simulink model "Autopilot_pwa_mdl"  (R2018b)
settings: Solver=VariableStepAuto  StartTime=0.0  StopTime=3  MaxStep=0.01  RelTol=1e-3
values from neighbouring files (symbols this model uses):
  ns = order(pdG)    [lpvctrl.m]    (also in lpvctrl_2.m = size(akh,1); pcss_Sfunction.m = order(sys))
  nu = length(pdG.InputGroup.ctrl)    [lpvctrl.m]    (also in lpvctrl_2.m; test_lpvanalysis.m = 0:10)
  ny = 0    [lft_pass.m]    (also in lft_pgss.m; lft_ppss.m; lpvctrl.m = length(pdG.OutputGroup.meas); lpvctrl_2.m = length(pdG.OutputGroup.meas))
  pdK = ppss(pdk,pdG.parset,                         'OutputName',pdG.OutputName(pdG.OutputGroup.meas),                         'InputName',pdG.InputName(pdG.InputGroup.ctrl))    [lpvctrl.m]    (also in lpvctrl_2.m)
libraries: cstblocks x4, simulink x1
settings Model: Creator=ferna  LastModifiedBy=ferna

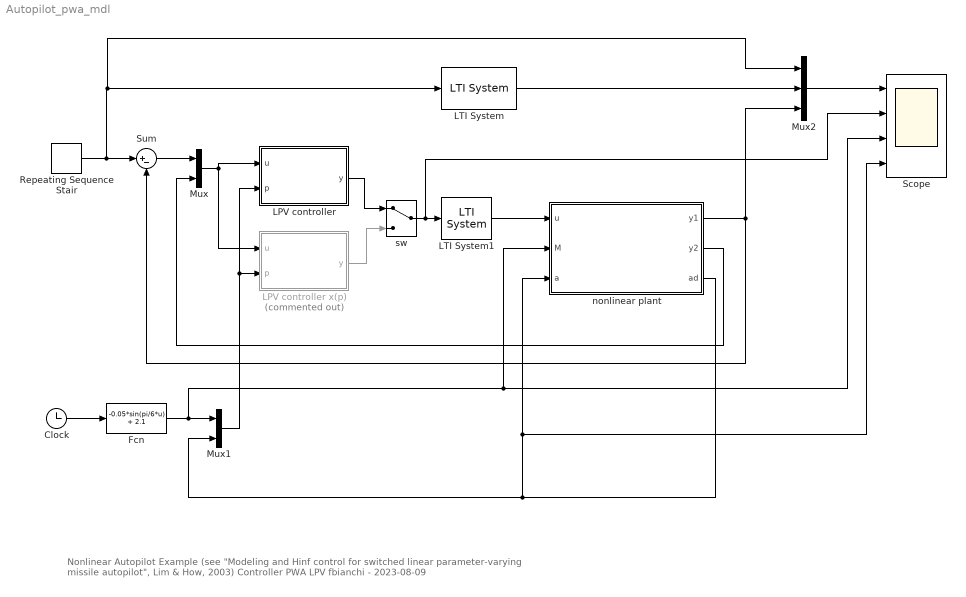
== system Autopilot_pwa_mdl ==
  note: Nonlinear Autopilot Example (see "Modeling and Hinf control for switched linear parameter-varying missile autopilot", Lim & How, 2003)
      | Controller PWA LPV
      | fbianchi - 2023-08-09
  Clock : Clock
  Fcn : Fcn  Expr=-0.05*sin(pi/6*u) + 2.1
  LPV controller : Subsystem  mask{pdG=pdK, x0=0}
      mask prompts: pdG "LPV Model (pass, ppss, pgss)"; x0 "Initial conditions"
      mask init:
      | % model dimensions
      | [ny,nu,ns,np,nv] = size(pdG);
      | 
      | % interpolation 
      | type = class(pdG);
      | switch type
      |     case 'pass'
      |         fcn = [];
      |         
      |     case 'pgss'
      |         fcn = pdg.parfcn;
      |         
      |     case 'ppss'
      |         fcn = pdG.parset;
      | end
      | 
      | % model matrices
      | M = [pdG.A pdG.B;
      |      pdG.C pdG.D];
      | Mdata = reshape(M,(ns+ny)*(ns+nu),nv,1);
      mask Display:
      | disp('LPV model')
      | port_label('input', 1, 'u')
      | port_label('input', 2, 'p')
      | port_label('output', 1, 'y')
  LPV controller x(p) : Subsystem  Commented=on  mask{pdK=pdK, x0=0}
      mask prompts: pdK "Controller (pcss)"; x0 "Initial conditions"
      mask init:
      | % model dimensions
      | [ny,nu,ns,np,nv] = size(pdK.ctrller);
      | 
      | % controller data
      | % interpolation 
      | type = class(pdK.ctrller);
      | switch type
      |     case 'pass'
      |         fcn = [];
      |         
      |     case 'pgss'
      |         fcn = pdK.ctrller.parfcn;
      |         
      |     case 'ppss'
      |         fcn = pdK.ctrller.parset;
      | end
      | 
      | % controller variables at p
      | K = [pdK.ctrller.A pdK.ctrller.B;
      |      pdK.ctrller.C pdK.ctrller.D];
      | Kdata = reshape(K,(ns+ny)*(ns+nu),nv,1);
      | 
      | % Lyapunov function at par
      | flagX = isnumeric(pdK.xFcn);
      | flagY = isnumeric(pdK.yFcn);
      | if (flagX == 0) && (flagY == 0)
      |     Ydata = reshape(pdK.yFcn.D,ns*ns,nv,1);
      |     Xdata = reshape(pdK.xFcn.D,ns*ns,nv,1);
      |     
      | elseif (flagX == 1) && (flagY == 0)
      |     Xdata = pdK.xFcn;
      |     Ydata = reshape(pdK.yFcn.D,ns*ns,nv,1);
      |     
      | elseif (flagX == 0) && (flagY == 1)
      |     Xdata = reshape(pdK.xFcn.D,ns*ns,nv,1);
      |     Ydata = pdK.yFcn;
      |     
      | end
      |                
      | % augmented plant matrices
      | Adata  = reshape(pdK.plant.A,ns*ns,nv,1);
      | b2 = pdK.plant.B(:,:,1);
      | c2 = pdK.plant.C(:,:,1);
      mask Display:
      | disp('pcss ctrller')
      | port_label('input', 1, 'u')
      | port_label('input', 2, 'p')
      | port_label('output', 1, 'y')
  LTI System : cstblocks/LTI System  sys=Wref  IC=[]
  LTI System1 : cstblocks/LTI System  sys=Act  IC=[]
  Mux : Mux  Inputs=2
  Mux1 : Mux  Inputs=2
  Mux2 : Mux  Inputs=3
  Repeating Sequence Stair : simulink/Sources/Repeating Sequence Stair  OutValues=[10 -15 0 0].'  tsamp=1  OutMin=[]  OutMax=[]  OutDataTypeStr=double  OutputDataTypeScalingMode=double  OutDataType=fixdt(0,8)  ConRadixGroup=Best Precision: Vector-wise  OutScaling=2^-12
  Scope : Scope  NumInputPorts=4
  Sum : Sum  Inputs=|+-
  nonlinear plant : Subsystem
  sw : ManualSwitch
  wires:
  LTI System1/1 -> nonlinear plant/1(u)
  Mux/1 -> LPV controller/1("u "), LPV controller x(p)/1("u ")
  Sum/1 -> Mux/1
  nonlinear plant/2(y2) -> Mux/2
  nonlinear plant/1(y1) -> Mux2/3, Sum/2
  Clock/1 -> Fcn/1
  Fcn/1 -> nonlinear plant/2(M), Scope/3, Mux1/1
  Mux1/1 -> LPV controller/2(p), LPV controller x(p)/2(p)
  Repeating Sequence Stair/1 -> LTI System/1, Mux2/1, Sum/1
  Mux2/1 -> Scope/1
  LTI System/1 -> Mux2/2
  nonlinear plant/3(ad) -> Mux1/2, nonlinear plant/3(a), Scope/4
  LPV controller/1(y) -> sw/1
  sw/1 -> Scope/2, LTI System1/1
  LPV controller x(p)/1(y) -> sw/2

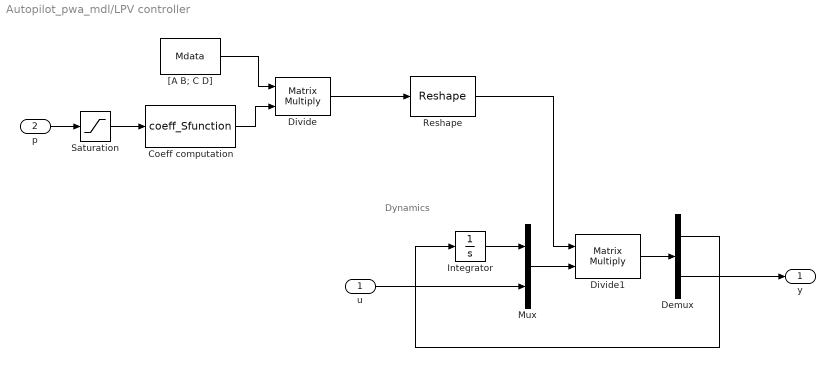
== system Autopilot_pwa_mdl/LPV controller ==
  note: Dynamics
  "u " : Inport
  p : Inport  Port=2
  Coeff computation : M-S-Function  FunctionName=coeff_Sfunction  Parameters=np, nv, fcn, type
  Demux : Demux  Outputs=[ns, ny]
  Divide : Product  Inputs=**  Multiplication=Matrix(*)
  Divide1 : Product  Inputs=**  Multiplication=Matrix(*)
  Integrator : Integrator
  Mux : Mux  Inputs=[ns, nu]
  Reshape : Reshape  OutputDimensionality=Customize  OutputDimensions=[ns+ny, ns+nu, 1]
  Saturation : Saturate  UpperLimit=pdK.parset.range(:,2)  LowerLimit=pdK.parset.range(:,1)
  "[A B; C D]" : Constant  Value=Mdata  VectorParams1D=off
  y : Outport
  wires:
  Divide/1 -> Reshape/1
  p/1 -> Saturation/1
  Saturation/1 -> Coeff computation/1
  Reshape/1 -> Divide1/1
  Mux/1 -> Divide1/2
  Divide1/1 -> Demux/1
  Demux/2 -> y/1
  Demux/1 -> Integrator/1
  Integrator/1 -> Mux/1
  "u "/1 -> Mux/2
  Coeff computation/1 -> Divide/2
  "[A B; C D]"/1 -> Divide/1

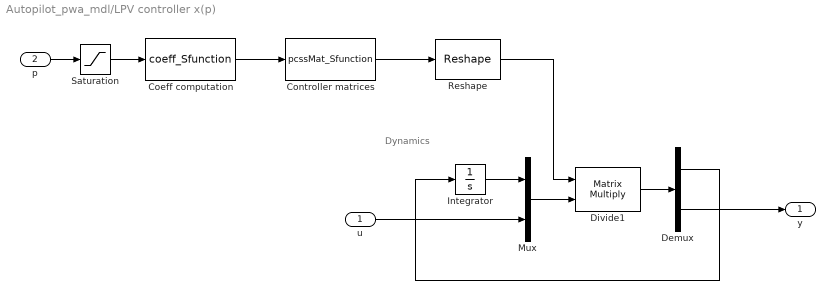
== system Autopilot_pwa_mdl/LPV controller x(p) ==
  note: Dynamics
  "u " : Inport
  p : Inport  Port=2
  Coeff computation : M-S-Function  FunctionName=coeff_Sfunction  Parameters=np, nv, fcn, type
  Controller matrices : M-S-Function  FunctionName=pcssMat_Sfunction  Parameters=Kdata, Xdata, Ydata, Adata, b2, c2, ns, ny, nu, nv, flagX, flagY
  Demux : Demux  Outputs=[ns, ny]
  Divide1 : Product  Inputs=**  Multiplication=Matrix(*)
  Integrator : Integrator
  Mux : Mux  Inputs=[ns, nu]
  Reshape : Reshape  OutputDimensionality=Customize  OutputDimensions=[ns+ny, ns+nu, 1]
  Saturation : Saturate  UpperLimit=pdK.parset.range(:,2)  LowerLimit=pdK.parset.range(:,1)
  y : Outport
  wires:
  "u "/1 -> Mux/2
  Integrator/1 -> Mux/1
  Demux/1 -> Integrator/1
  Demux/2 -> y/1
  Divide1/1 -> Demux/1
  Mux/1 -> Divide1/2
  Reshape/1 -> Divide1/1
  Saturation/1 -> Coeff computation/1
  p/1 -> Saturation/1
  Coeff computation/1 -> Controller matrices/1
  Controller matrices/1 -> Reshape/1

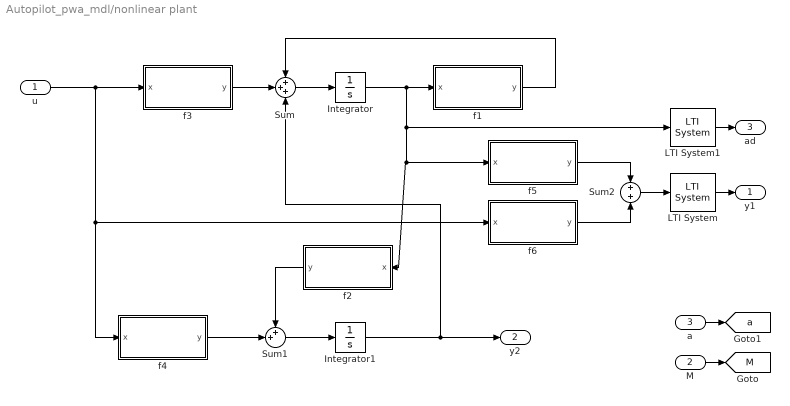
== system Autopilot_pwa_mdl/nonlinear plant ==
  u : Inport
  M : Inport  Port=2
  a : Inport  Port=3
  Integrator : Integrator
  Integrator1 : Integrator
  LTI System : cstblocks/LTI System  sys=F  IC=[]
  LTI System1 : cstblocks/LTI System  sys=F  IC=[]
  Sum : Sum  Inputs=+++
  Sum1 : Sum  Inputs=++|
  Sum2 : Sum
  f1 : Subsystem
  f2 : Subsystem
  f3 : Subsystem
  f4 : Subsystem
  f5 : Subsystem
  f6 : Subsystem
  y1 : Outport
  y2 : Outport  Port=2
  ad : Outport  Port=3
  tag scope: M=global, a=global
  wires:
  a/1 -> [a]
  f6/1(y) -> Sum2/2
  M/1 -> [M]
  f1/1(y) -> Sum/1
  f3/1(y) -> Sum/2
  Integrator/1 -> f2/1(x), f5/1(x), LTI System1/1, f1/1(x)
  Integrator1/1 -> Sum/3, y2/1
  f5/1(y) -> Sum2/1
  Sum/1 -> Integrator/1
  Sum2/1 -> LTI System/1
  u/1 -> f6/1(x), f4/1(x), f3/1(x)
  LTI System/1 -> y1/1
  LTI System1/1 -> ad/1
  Sum1/1 -> Integrator1/1
  f4/1(y) -> Sum1/2
  f2/1(y) -> Sum1/1

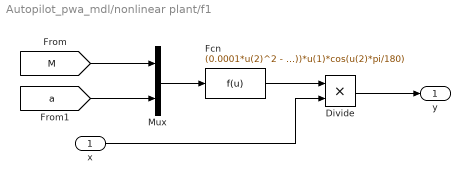
== system Autopilot_pwa_mdl/nonlinear plant/f1 ==
  x : Inport
  Divide : Product  Inputs=**
  Fcn : Fcn  Expr=(0.0001*u(2)^2 - 0.0112*abs(u(2)) - 0.2010*(2 - u(1)/3))*u(1)*cos(u(2)*pi/180)
  Mux : Mux  Inputs=2
  y : Outport
  wires:
  [a] -> Mux/2
  Mux/1 -> Fcn/1
  [M] -> Mux/1
  Fcn/1 -> Divide/1
  Divide/1 -> y/1
  x/1 -> Divide/2

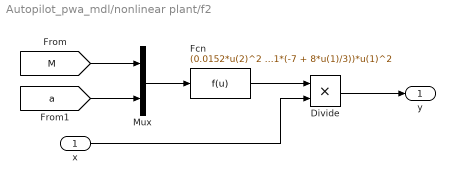
== system Autopilot_pwa_mdl/nonlinear plant/f2 ==
  x : Inport
  Divide : Product  Inputs=**
  Fcn : Fcn  Expr=(0.0152*u(2)^2 - 1.3765*abs(u(2)) + 3.6001*(-7 + 8*u(1)/3))*u(1)^2
  Mux : Mux  Inputs=2
  y : Outport
  wires:
  x/1 -> Divide/2
  Divide/1 -> y/1
  Fcn/1 -> Divide/1
  [M] -> Mux/1
  Mux/1 -> Fcn/1
  [a] -> Mux/2

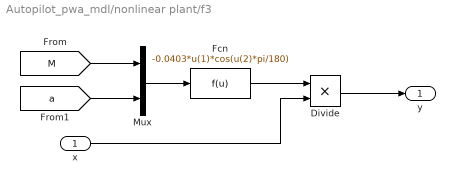
== system Autopilot_pwa_mdl/nonlinear plant/f3 ==
  x : Inport
  Divide : Product  Inputs=**
  Fcn : Fcn  Expr=-0.0403*u(1)*cos(u(2)*pi/180)
  Mux : Mux  Inputs=2
  y : Outport
  wires:
  Mux/1 -> Fcn/1
  Fcn/1 -> Divide/1
  Divide/1 -> y/1
  x/1 -> Divide/2
  [a] -> Mux/2
  [M] -> Mux/1

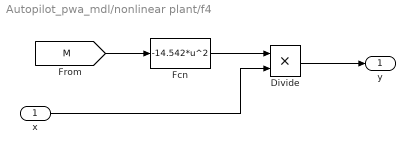
== system Autopilot_pwa_mdl/nonlinear plant/f4 ==
  x : Inport
  Divide : Product  Inputs=**
  Fcn : Fcn  Expr=-14.542*u^2
  y : Outport
  wires:
  x/1 -> Divide/2
  Divide/1 -> y/1
  Fcn/1 -> Divide/1
  [M] -> Fcn/1

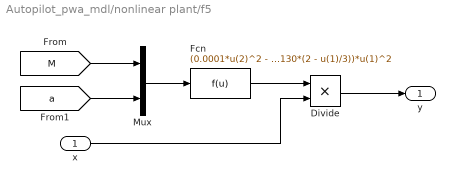
== system Autopilot_pwa_mdl/nonlinear plant/f5 ==
  x : Inport
  Divide : Product  Inputs=**
  Fcn : Fcn  Expr=(0.0001*u(2)^2 - 0.0063*abs(u(2)) - 0.1130*(2 - u(1)/3))*u(1)^2
  Mux : Mux  Inputs=2
  y : Outport
  wires:
  Mux/1 -> Fcn/1
  Fcn/1 -> Divide/1
  Divide/1 -> y/1
  x/1 -> Divide/2
  [a] -> Mux/2
  [M] -> Mux/1

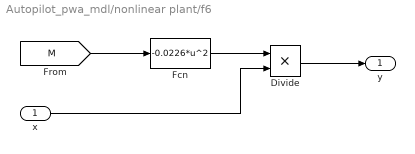
== system Autopilot_pwa_mdl/nonlinear plant/f6 ==
  x : Inport
  Divide : Product  Inputs=**
  Fcn : Fcn  Expr=-0.0226*u^2
  y : Outport
  wires:
  x/1 -> Divide/2
  Divide/1 -> y/1
  Fcn/1 -> Divide/1
  [M] -> Fcn/1
